simulink model "verify_ValveTable_mdl"  (R2016b)
settings: Solver=ode45  StartTime=0.0  StopTime=75  MaxStep=1  RelTol=1e-3  EnableMultiTasking=on
undefined symbols (not defined in the file or in its folder): DPConstant, DPLinear, DPQuadratic, path_carnot, Pressure
libraries: carnot x2, simulink x1
settings Model: Creator=drhf  LastModifiedBy=drhf
settings DataIOCC: SaveFormat=Array  SignalLoggingSaveFormat=ModelDataLogs
settings OptimizationCC: ExpressionDepthLimit=2147483647  LifeSpan=inf
settings DebuggingCC: UnderspecifiedInitializationDetection=Classic  MergeDetectMultiDrivingBlocksExec=none  SolverPrmCheckMsg=warning  FcnCallInpInsideContextMsg=warning  StateNameClashWarn=warning  SFUnexpectedBacktrackingDiag=warning  SFNoUnconditionalDefaultTransitionDiag=warning  SFExecutionAtInitializationDiag=none
settings HardwareCC: ProdBitPerPointer=32  ProdBitPerSizeT=32  ProdBitPerPtrDiffT=32  ProdLargestAtomicFloat=None  ProdIntDivRoundTo=Undefined  ProdEndianess=Unspecified  ProdWordSize=32  ProdHWDeviceType=32-bit Generic
settings ModelReferenceCC: PropagateSignalLabelsOutOfModel=off
settings GRTTargetCC: TargetLangStandard=C89/C90 (ANSI)  GeneratePreprocessorConditionals=Disable all  CombineOutputUpdateFcns=off  GRTInterface=on
settings ConfigComp: CovMetricSettings=dw  CovHtmlReporting=on  CovSaveCumulativeToWorkspaceVar=on  CovSaveSingleToWorkspaceVar=on  CovExternalEMLEnable=off

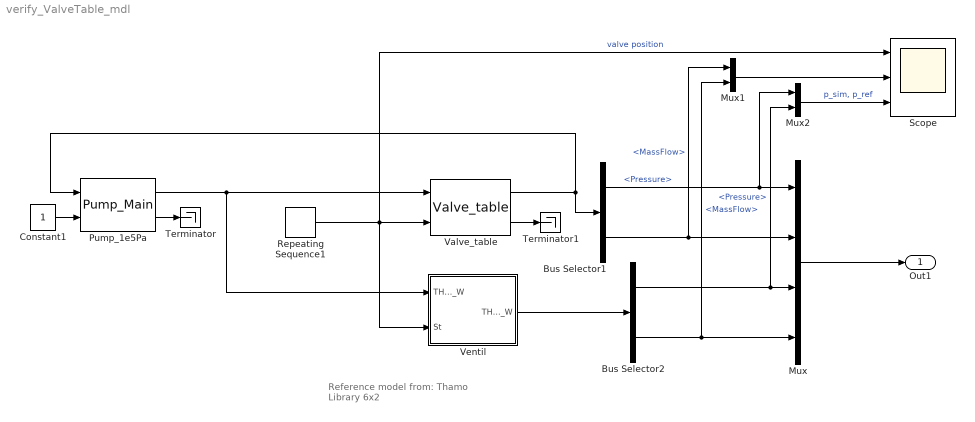
== system verify_ValveTable_mdl ==
  note: Reference model from:
      | Thamo Library 6x2
  Bus Selector1 : BusSelector  OutputSignals=Pressure,MassFlow
  Bus Selector2 : BusSelector  OutputSignals=Pressure,MassFlow
  Constant1 : Constant
  Mux : Mux
  Mux1 : Mux  Inputs=2
  Mux2 : Mux  Inputs=2
  Pump_1e5Pa : carnot/Hydraulics/Pump_Main  Tini=20  p0=3e5  IDpreset=pressure drop  fluid=Water  mix=0  mix2=0  mix3=0  t1=0.01  PathName=fullfile(path_carnot('libsl'), 'Hydraulics', 'Pump_Main', 'parameter_set')  FileName='Pump6m.mat'  userPath=off  userParam=off  a0=60000  a1=-43200  a2=0  dia=0.025  UA=1  mcp=4182  e0=50  e1=28.8  e2=-10.368
  Repeating Sequence1 : simulink/Sources/Repeating Sequence  rep_seq_t=[0 20 60 80]  rep_seq_y=[1 1 0 0]
  Scope : Scope  NumInputPorts=3
  Terminator : Terminator
  Terminator1 : Terminator
  Valve_table : carnot/Hydraulics/Valve_table  h=[0 1]  psi=[0.04 1]  kvs=0.9  dt_V=0.01
  Ventil : Subsystem  mask(Ventil){ART=linear, kvs=0.9, n_0=0.04, dt_V=0.01}
      mask prompts: ART "Ventilcharakteristik"; kvs "kvs-Wert in m³/s"; n_0 "Rel. Durchflusskoeffizient"; dt_V "Ventillaufzeit in s"
      mask Help: web(fullfile(path_carnot('help'),'Valve.html'),'-helpbrowser')
      mask TypeOptions ART: linear | gleichprozentig
      mask Callback ART:
      | ART=1;
      | ART=2;
      mask Display: plot(0,10,120,180,[30,70,70,30,30]*0.8,[60,40,60,40,60]*0.8,[60,40]*0.8,[80,80]*0.8,[50,50]*0.8,[50,80]*0.8)
  Out1 : Outport
  wires:
  Mux/1 -> Out1/1
  Bus Selector1/1 -> Mux2/1, Mux/1  "<Pressure>"
  Bus Selector1/2 -> Mux1/1, Mux/2  "<MassFlow>"
  Valve_table/1 -> Bus Selector1/1, Pump_1e5Pa/1
  Repeating Sequence1/1 -> Ventil/2(St), Valve_table/2, Scope/1  "valve position"
  Pump_1e5Pa/1 -> Valve_table/1, Ventil/1(THB__1_W)
  Ventil/1(THB__2_W) -> Bus Selector2/1
  Bus Selector2/1 -> Mux2/2, Mux/3  "<Pressure>"
  Mux2/1 -> Scope/3  "p_sim, p_ref"
  Constant1/1 -> Pump_1e5Pa/2
  Pump_1e5Pa/2 -> Terminator/1
  Bus Selector2/2 -> Mux1/2, Mux/4  "<MassFlow>"
  Mux1/1 -> Scope/2
  Valve_table/2 -> Terminator1/1

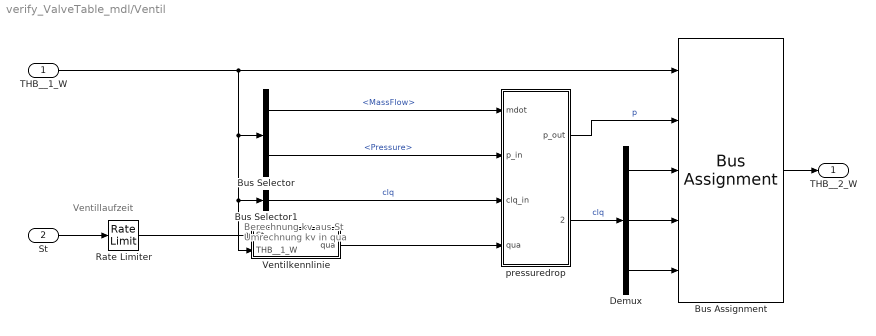
== system verify_ValveTable_mdl/Ventil ==
  note: Ventillaufzeit
  note: Berechnung kv aus St
      | Umrechnung kv in qua
  THB__1_W : Inport
  St : Inport  Port=2
  Bus Assignment : BusAssignment  AssignedSignals=Pressure,DPConstant,DPLinear,DPQuadratic
  Bus Selector : BusSelector  OutputSignals=MassFlow,Pressure
  Bus Selector1 : BusSelector  OutputSignals=DPConstant,DPLinear,DPQuadratic  OutputAsBus=on
  Demux : Demux  Outputs=3
  Rate Limiter : RateLimiter  RisingSlewLimit=1/dt_V  FallingSlewLimit=-1/dt_V  SampleTimeMode=inherited
  Ventilkennlinie : Subsystem
  pressuredrop : Subsystem  mask(pressure drop){}
      mask help:
      | Pressure drop according to input values of con, lin and qua:
      | dp = con + lin*mdot + qua*mdot²
      | The coefficients are also added to the correponding THB elements.
      mask Help: web(fullfile(path_carnot('help'),'Pressuredrop.html'),'-helpbrowser')
  THB__2_W : Outport
  wires:
  Demux/3 -> Bus Assignment/5
  Demux/2 -> Bus Assignment/4
  Bus Selector1/1 -> pressuredrop/3(clq_in)  "clq"
  pressuredrop/1(p_out) -> Bus Assignment/2  "p"
  Bus Selector/1 -> pressuredrop/1(mdot)  "<MassFlow>"
  Bus Selector/2 -> pressuredrop/2(p_in)  "<Pressure>"
  pressuredrop/2(clq_out) -> Demux/1  "clq"
  St/1 -> Rate Limiter/1
  THB__1_W/1 -> Bus Selector1/1, Ventilkennlinie/2(THB__1_W), Bus Selector/1, Bus Assignment/1
  Bus Assignment/1 -> THB__2_W/1
  Demux/1 -> Bus Assignment/3
  Ventilkennlinie/1(qua) -> pressuredrop/4(qua)
  Rate Limiter/1 -> Ventilkennlinie/1(St)

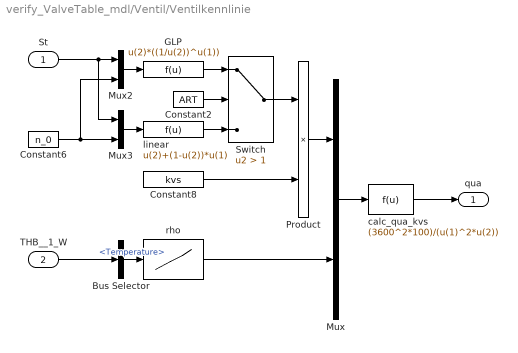
== system verify_ValveTable_mdl/Ventil/Ventilkennlinie ==
  St : Inport
  THB__1_W : Inport  Port=2
  Bus Selector : BusSelector  OutputSignals=Temperature
  Constant2 : Constant  Value=ART
  Constant6 : Constant  Value=n_0
  Constant8 : Constant  Value=kvs
  GLP : Fcn  Expr=u(2)*((1/u(2))^u(1))
  Mux : Mux  Inputs=2
  Mux2 : Mux  Inputs=2
  Mux3 : Mux  Inputs=2
  Product : Product
  Switch : Switch  Criteria=u2 > Threshold  Threshold=1
  calc_qua_kvs : Fcn  Expr=(3600^2*100)/(u(1)^2*u(2))
  linear : Fcn  Expr=u(2)+(1-u(2))*u(1)
  rho : Lookup_n-D  NumberOfTableDimensions=1  BreakpointsForDimension1=[0,10,20,30,40,50,60,70,80,90,100]  Table=[999.84,999.7,998.2,995.64,992.21,988.03,983.19,977.76,971.79,965.3,958.35]  InternalRulePriority=Speed  RndMeth=Simplest  InputSameDT=on
  qua : Outport
  wires:
  Bus Selector/1 -> rho/1  "<Temperature>"
  St/1 -> Mux2/1, Mux3/1
  linear/1 -> Switch/3
  Mux2/1 -> GLP/1
  Mux3/1 -> linear/1
  Constant6/1 -> Mux2/2, Mux3/2
  Constant8/1 -> Product/2
  Switch/1 -> Product/1
  Constant2/1 -> Switch/2
  GLP/1 -> Switch/1
  THB__1_W/1 -> Bus Selector/1
  calc_qua_kvs/1 -> qua/1
  Mux/1 -> calc_qua_kvs/1
  Product/1 -> Mux/1
  rho/1 -> Mux/2

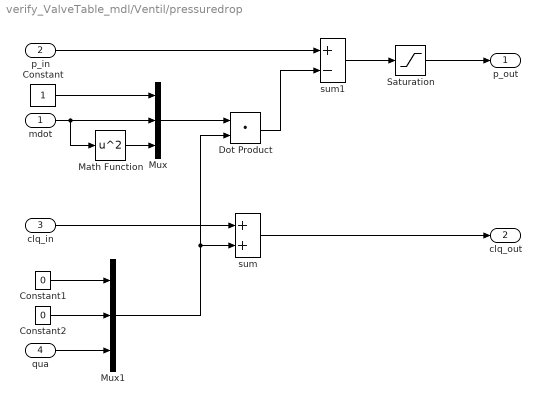
== system verify_ValveTable_mdl/Ventil/pressuredrop ==
  mdot : Inport
  p_in : Inport  Port=2
  clq_in : Inport  Port=3
  qua : Inport  Port=4
  Constant : Constant
  Constant1 : Constant  Value=0
  Constant2 : Constant  Value=0
  Dot Product : DotProduct  InputSameDT=on  OutDataTypeStr=Inherit: Inherit via internal rule
  Math Function : Math  Operator=square  SaturateOnIntegerOverflow=on
  Mux : Mux  Inputs=3
  Mux1 : Mux  Inputs=3
  Saturation : Saturate  UpperLimit=inf  LowerLimit=0
  sum : Sum  SaturateOnIntegerOverflow=on  InputSameDT=on  OutDataTypeStr=Inherit: Same as first input
  sum1 : Sum  Inputs=+-  SaturateOnIntegerOverflow=on  InputSameDT=on  OutDataTypeStr=Inherit: Same as first input
  p_out : Outport
  clq_out : Outport  Port=2
  wires:
  Saturation/1 -> p_out/1
  Constant/1 -> Mux/1
  mdot/1 -> Mux/2, Math Function/1
  Math Function/1 -> Mux/3
  Mux/1 -> Dot Product/1
  qua/1 -> Mux1/3
  clq_in/1 -> sum/1
  sum/1 -> clq_out/1
  Mux1/1 -> sum/2, Dot Product/2
  Dot Product/1 -> sum1/2
  p_in/1 -> sum1/1
  sum1/1 -> Saturation/1
  Constant1/1 -> Mux1/1
  Constant2/1 -> Mux1/2
